simulink model "merge_activation"  (Simulink 8.2)
settings: Solver=ode1  StartTime=0.0  StopTime=Inf  FixedStep=0.001  RelTol=1e-3
PostLoadFcn:
  | , if any(exist('dsrtsu_mdlpostloadfcn', 'file') == [2, 3, 6]), try dsrtsu_mdlpostloadfcn('Execute', bdroot); catch fprintf('Error in PostLoadFcn (dsrtsu_mdlpostloadfcn) for model "%s":\n %s\n', bdroot, lasterr); end, end,
settings Model: DSRTSU_INTERNAL_RTI_VER=450  DSRTSU_INTERNAL_RTI_TYPE=rti1401  DSRTSU_INTERNAL_RTIFPGA=40  Creator=rushk1  LastModifiedBy=rushk1  BufferReuse=off
settings DataIOCC: SignalLoggingSaveFormat=Dataset
settings OptimizationCC: BlockReduction=off  OptimizeBlockIOStorage=off  BufferReuse=off  ExpressionFolding=off  ExpressionDepthLimit=128  LocalBlockOutputs=off
settings DebuggingCC: FcnCallInpInsideContextMsg=EnableAllAsError  StateNameClashWarn=none
settings HardwareCC: TargetHWDeviceType=Generic->Custom
settings RTWCC: SystemTargetFile=rti1401.tlc  MakeCommand=make_rti  TemplateMakefile=rti1401.tmf  Description=dSPACE DS1401 Hardware Platform  ProcessScript=rti1401_make_rtw_hook
settings STFCustomTargetCC: CodeReplacementLibrary=ANSI_C  ParMdlRefBuildCompliant=on  GeneratePreprocessorConditionals=Disable all  MatFileLogging=on  SystemTargetFile=rti1401.tlc
settings GRTTargetCC: CompOptLevelCompliant=off  ConcurrentExecutionCompliant=off  ExtModeMexFile=noextcomm
settings CustomProperty: DataType=RTWOptions_EnumType_C__Program Files_dSPACE RCPHIL 2014-B_MATLAB_RTI_RTI1401_TLC_rti1401_1InitialSimState  Value=RUN
settings EnumStrPairs: String=RUN

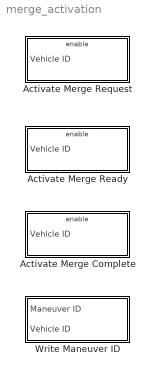
== system merge_activation ==
  Activate Merge Complete : Subsystem
  Activate Merge Ready : Subsystem
  Activate Merge Request : Subsystem
  Write Maneuver ID : Subsystem

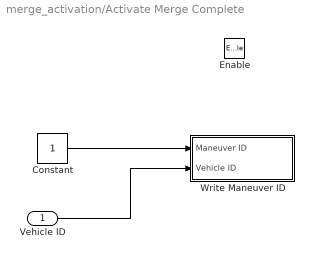
== system merge_activation/Activate Merge Complete ==
  Vehicle ID : Inport
  Enable : EnablePort
  Constant : Constant
  Write Maneuver ID : Subsystem
  wires:
  Constant/1 -> Write Maneuver ID/1(Maneuver ID)
  Vehicle ID/1 -> Write Maneuver ID/2(Vehicle ID)

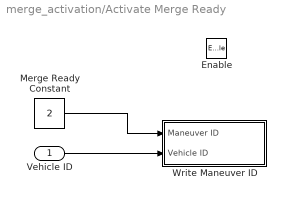
== system merge_activation/Activate Merge Ready ==
  Vehicle ID : Inport
  Enable : EnablePort
  Merge Ready Constant : Constant  Value=2
  Write Maneuver ID : Subsystem
  wires:
  Vehicle ID/1 -> Write Maneuver ID/2(Vehicle ID)
  Merge Ready Constant/1 -> Write Maneuver ID/1(Maneuver ID)

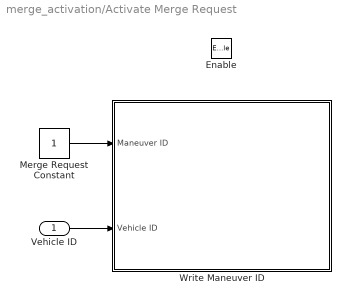
== system merge_activation/Activate Merge Request ==
  Vehicle ID : Inport
  Enable : EnablePort
  Merge Request Constant : Constant
  Write Maneuver ID : Subsystem
  wires:
  Merge Request Constant/1 -> Write Maneuver ID/1(Maneuver ID)
  Vehicle ID/1 -> Write Maneuver ID/2(Vehicle ID)

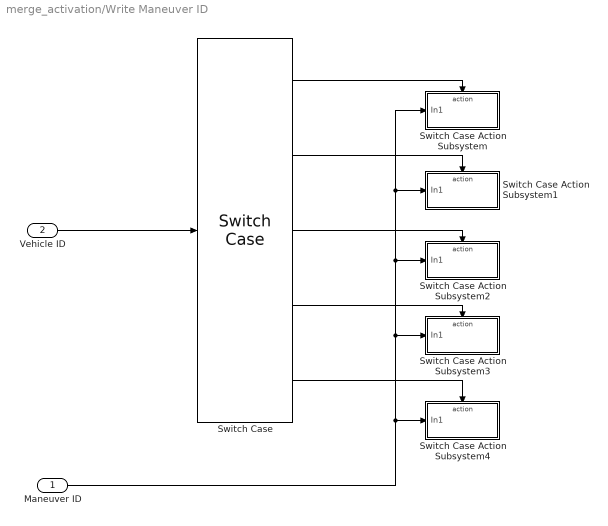
== system merge_activation/Write Maneuver ID ==
  Maneuver ID : Inport
  Vehicle ID : Inport  Port=2
  Switch Case : SwitchCase  CaseConditions={1,2,3,4,5}  ShowDefaultCase=off
  Switch Case Action Subsystem : Subsystem  TreatAsAtomicUnit=on
  Switch Case Action Subsystem1 : Subsystem  TreatAsAtomicUnit=on
  Switch Case Action Subsystem2 : Subsystem  TreatAsAtomicUnit=on
  Switch Case Action Subsystem3 : Subsystem  TreatAsAtomicUnit=on
  Switch Case Action Subsystem4 : Subsystem  TreatAsAtomicUnit=on
  wires:
  Switch Case/5 -> Switch Case Action Subsystem4/Action
  Switch Case/4 -> Switch Case Action Subsystem3/Action
  Switch Case/3 -> Switch Case Action Subsystem2/Action
  Switch Case/2 -> Switch Case Action Subsystem1/Action
  Switch Case/1 -> Switch Case Action Subsystem/Action
  Vehicle ID/1 -> Switch Case/1
  Maneuver ID/1 -> Switch Case Action Subsystem/1(In1), Switch Case Action Subsystem1/1(In1), Switch Case Action Subsystem2/1(In1), Switch Case Action Subsystem3/1(In1), Switch Case Action Subsystem4/1(In1)

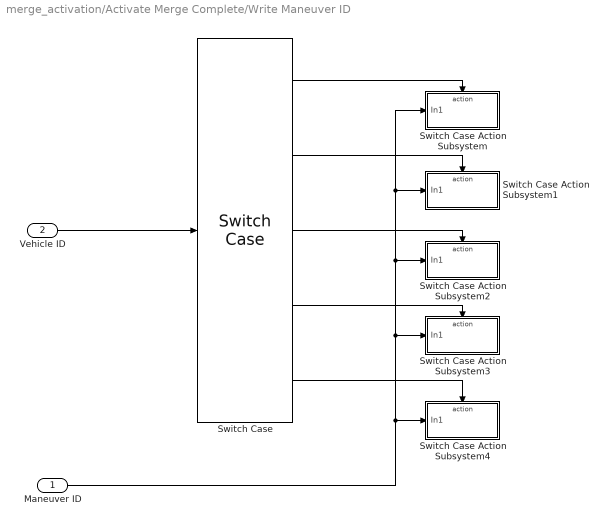
== system merge_activation/Activate Merge Complete/Write Maneuver ID ==
  Maneuver ID : Inport
  Vehicle ID : Inport  Port=2
  Switch Case : SwitchCase  CaseConditions={1,2,3,4,5}  ShowDefaultCase=off
  Switch Case Action Subsystem : Subsystem  TreatAsAtomicUnit=on
  Switch Case Action Subsystem1 : Subsystem  TreatAsAtomicUnit=on
  Switch Case Action Subsystem2 : Subsystem  TreatAsAtomicUnit=on
  Switch Case Action Subsystem3 : Subsystem  TreatAsAtomicUnit=on
  Switch Case Action Subsystem4 : Subsystem  TreatAsAtomicUnit=on
  wires:
  Switch Case/5 -> Switch Case Action Subsystem4/Action
  Switch Case/4 -> Switch Case Action Subsystem3/Action
  Switch Case/3 -> Switch Case Action Subsystem2/Action
  Switch Case/2 -> Switch Case Action Subsystem1/Action
  Switch Case/1 -> Switch Case Action Subsystem/Action
  Vehicle ID/1 -> Switch Case/1
  Maneuver ID/1 -> Switch Case Action Subsystem/1(In1), Switch Case Action Subsystem1/1(In1), Switch Case Action Subsystem2/1(In1), Switch Case Action Subsystem3/1(In1), Switch Case Action Subsystem4/1(In1)

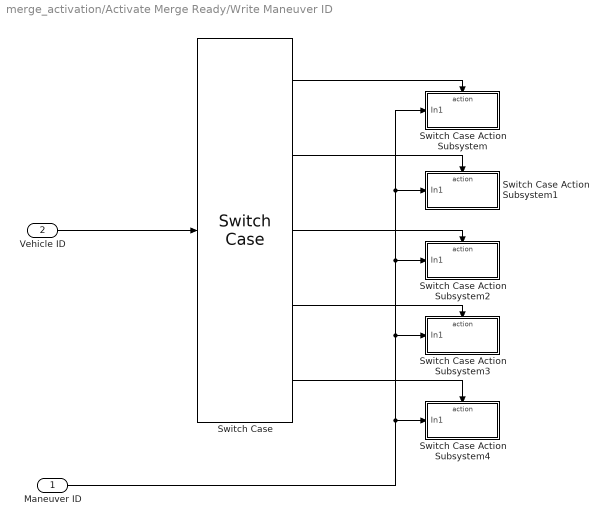
== system merge_activation/Activate Merge Ready/Write Maneuver ID ==
  Maneuver ID : Inport
  Vehicle ID : Inport  Port=2
  Switch Case : SwitchCase  CaseConditions={1,2,3,4,5}  ShowDefaultCase=off
  Switch Case Action Subsystem : Subsystem  TreatAsAtomicUnit=on
  Switch Case Action Subsystem1 : Subsystem  TreatAsAtomicUnit=on
  Switch Case Action Subsystem2 : Subsystem  TreatAsAtomicUnit=on
  Switch Case Action Subsystem3 : Subsystem  TreatAsAtomicUnit=on
  Switch Case Action Subsystem4 : Subsystem  TreatAsAtomicUnit=on
  wires:
  Switch Case/5 -> Switch Case Action Subsystem4/Action
  Switch Case/4 -> Switch Case Action Subsystem3/Action
  Switch Case/3 -> Switch Case Action Subsystem2/Action
  Switch Case/2 -> Switch Case Action Subsystem1/Action
  Switch Case/1 -> Switch Case Action Subsystem/Action
  Vehicle ID/1 -> Switch Case/1
  Maneuver ID/1 -> Switch Case Action Subsystem/1(In1), Switch Case Action Subsystem1/1(In1), Switch Case Action Subsystem2/1(In1), Switch Case Action Subsystem3/1(In1), Switch Case Action Subsystem4/1(In1)

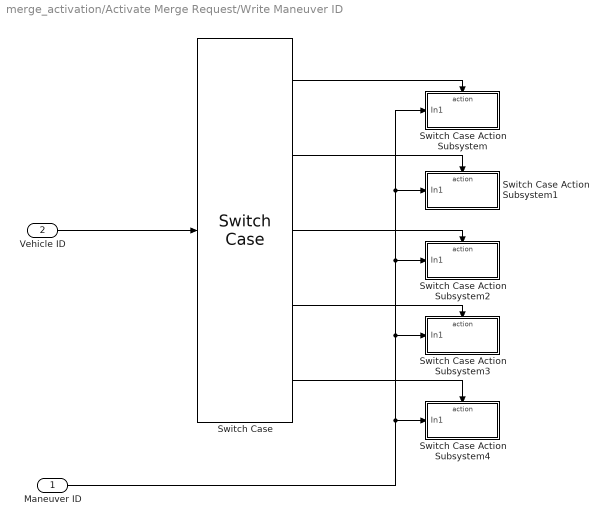
== system merge_activation/Activate Merge Request/Write Maneuver ID ==
  Maneuver ID : Inport
  Vehicle ID : Inport  Port=2
  Switch Case : SwitchCase  CaseConditions={1,2,3,4,5}  ShowDefaultCase=off
  Switch Case Action Subsystem : Subsystem  TreatAsAtomicUnit=on
  Switch Case Action Subsystem1 : Subsystem  TreatAsAtomicUnit=on
  Switch Case Action Subsystem2 : Subsystem  TreatAsAtomicUnit=on
  Switch Case Action Subsystem3 : Subsystem  TreatAsAtomicUnit=on
  Switch Case Action Subsystem4 : Subsystem  TreatAsAtomicUnit=on
  wires:
  Switch Case/5 -> Switch Case Action Subsystem4/Action
  Switch Case/4 -> Switch Case Action Subsystem3/Action
  Switch Case/3 -> Switch Case Action Subsystem2/Action
  Switch Case/2 -> Switch Case Action Subsystem1/Action
  Switch Case/1 -> Switch Case Action Subsystem/Action
  Vehicle ID/1 -> Switch Case/1
  Maneuver ID/1 -> Switch Case Action Subsystem/1(In1), Switch Case Action Subsystem1/1(In1), Switch Case Action Subsystem2/1(In1), Switch Case Action Subsystem3/1(In1), Switch Case Action Subsystem4/1(In1)

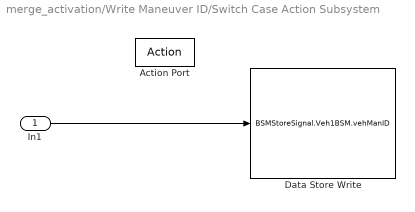
== system merge_activation/Write Maneuver ID/Switch Case Action Subsystem ==
  In1 : Inport
  Action Port : ActionPort
  Data Store Write : DataStoreWrite  DataStoreName=BSMStoreSignal  DataStoreElements=BSMStoreSignal.Veh1BSM.vehManID
  wires:
  In1/1 -> Data Store Write/1

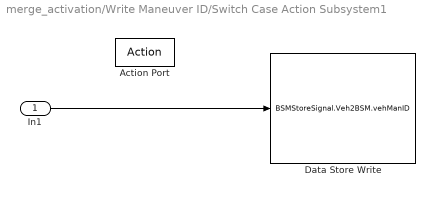
== system merge_activation/Write Maneuver ID/Switch Case Action Subsystem1 ==
  In1 : Inport
  Action Port : ActionPort
  Data Store Write : DataStoreWrite  DataStoreName=BSMStoreSignal  DataStoreElements=BSMStoreSignal.Veh2BSM.vehManID
  wires:
  In1/1 -> Data Store Write/1

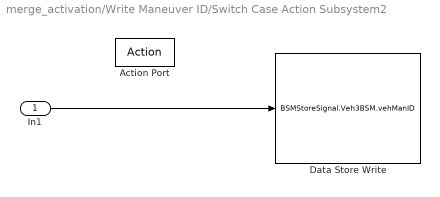
== system merge_activation/Write Maneuver ID/Switch Case Action Subsystem2 ==
  In1 : Inport
  Action Port : ActionPort
  Data Store Write : DataStoreWrite  DataStoreName=BSMStoreSignal  DataStoreElements=BSMStoreSignal.Veh3BSM.vehManID
  wires:
  In1/1 -> Data Store Write/1

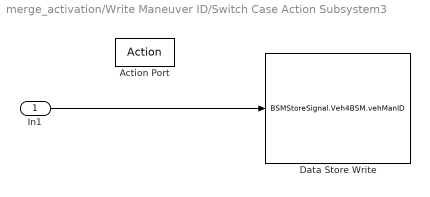
== system merge_activation/Write Maneuver ID/Switch Case Action Subsystem3 ==
  In1 : Inport
  Action Port : ActionPort
  Data Store Write : DataStoreWrite  DataStoreName=BSMStoreSignal  DataStoreElements=BSMStoreSignal.Veh4BSM.vehManID
  wires:
  In1/1 -> Data Store Write/1

== system merge_activation/Write Maneuver ID/Switch Case Action Subsystem4 ==
  In1 : Inport
  Action Port : ActionPort
  Data Store Write : DataStoreWrite  DataStoreName=BSMStoreSignal  DataStoreElements=BSMStoreSignal.Veh5BSM.vehManID
  wires:
  In1/1 -> Data Store Write/1

== system merge_activation/Activate Merge Complete/Write Maneuver ID/Switch Case Action Subsystem ==
  In1 : Inport
  Action Port : ActionPort
  Data Store Write : DataStoreWrite  DataStoreName=BSMStoreSignal  DataStoreElements=BSMStoreSignal.Veh1BSM.vehManID
  wires:
  In1/1 -> Data Store Write/1

== system merge_activation/Activate Merge Complete/Write Maneuver ID/Switch Case Action Subsystem1 ==
  In1 : Inport
  Action Port : ActionPort
  Data Store Write : DataStoreWrite  DataStoreName=BSMStoreSignal  DataStoreElements=BSMStoreSignal.Veh2BSM.vehManID
  wires:
  In1/1 -> Data Store Write/1

== system merge_activation/Activate Merge Complete/Write Maneuver ID/Switch Case Action Subsystem2 ==
  In1 : Inport
  Action Port : ActionPort
  Data Store Write : DataStoreWrite  DataStoreName=BSMStoreSignal  DataStoreElements=BSMStoreSignal.Veh3BSM.vehManID
  wires:
  In1/1 -> Data Store Write/1

== system merge_activation/Activate Merge Complete/Write Maneuver ID/Switch Case Action Subsystem3 ==
  In1 : Inport
  Action Port : ActionPort
  Data Store Write : DataStoreWrite  DataStoreName=BSMStoreSignal  DataStoreElements=BSMStoreSignal.Veh4BSM.vehManID
  wires:
  In1/1 -> Data Store Write/1

== system merge_activation/Activate Merge Complete/Write Maneuver ID/Switch Case Action Subsystem4 ==
  In1 : Inport
  Action Port : ActionPort
  Data Store Write : DataStoreWrite  DataStoreName=BSMStoreSignal  DataStoreElements=BSMStoreSignal.Veh5BSM.vehManID
  wires:
  In1/1 -> Data Store Write/1

== system merge_activation/Activate Merge Ready/Write Maneuver ID/Switch Case Action Subsystem ==
  In1 : Inport
  Action Port : ActionPort
  Data Store Write : DataStoreWrite  DataStoreName=BSMStoreSignal  DataStoreElements=BSMStoreSignal.Veh1BSM.vehManID
  wires:
  In1/1 -> Data Store Write/1

== system merge_activation/Activate Merge Ready/Write Maneuver ID/Switch Case Action Subsystem1 ==
  In1 : Inport
  Action Port : ActionPort
  Data Store Write : DataStoreWrite  DataStoreName=BSMStoreSignal  DataStoreElements=BSMStoreSignal.Veh2BSM.vehManID
  wires:
  In1/1 -> Data Store Write/1

== system merge_activation/Activate Merge Ready/Write Maneuver ID/Switch Case Action Subsystem2 ==
  In1 : Inport
  Action Port : ActionPort
  Data Store Write : DataStoreWrite  DataStoreName=BSMStoreSignal  DataStoreElements=BSMStoreSignal.Veh3BSM.vehManID
  wires:
  In1/1 -> Data Store Write/1

== system merge_activation/Activate Merge Ready/Write Maneuver ID/Switch Case Action Subsystem3 ==
  In1 : Inport
  Action Port : ActionPort
  Data Store Write : DataStoreWrite  DataStoreName=BSMStoreSignal  DataStoreElements=BSMStoreSignal.Veh4BSM.vehManID
  wires:
  In1/1 -> Data Store Write/1

== system merge_activation/Activate Merge Ready/Write Maneuver ID/Switch Case Action Subsystem4 ==
  In1 : Inport
  Action Port : ActionPort
  Data Store Write : DataStoreWrite  DataStoreName=BSMStoreSignal  DataStoreElements=BSMStoreSignal.Veh5BSM.vehManID
  wires:
  In1/1 -> Data Store Write/1

== system merge_activation/Activate Merge Request/Write Maneuver ID/Switch Case Action Subsystem ==
  In1 : Inport
  Action Port : ActionPort
  Data Store Write : DataStoreWrite  DataStoreName=BSMStoreSignal  DataStoreElements=BSMStoreSignal.Veh1BSM.vehManID
  wires:
  In1/1 -> Data Store Write/1

== system merge_activation/Activate Merge Request/Write Maneuver ID/Switch Case Action Subsystem1 ==
  In1 : Inport
  Action Port : ActionPort
  Data Store Write : DataStoreWrite  DataStoreName=BSMStoreSignal  DataStoreElements=BSMStoreSignal.Veh2BSM.vehManID
  wires:
  In1/1 -> Data Store Write/1

== system merge_activation/Activate Merge Request/Write Maneuver ID/Switch Case Action Subsystem2 ==
  In1 : Inport
  Action Port : ActionPort
  Data Store Write : DataStoreWrite  DataStoreName=BSMStoreSignal  DataStoreElements=BSMStoreSignal.Veh3BSM.vehManID
  wires:
  In1/1 -> Data Store Write/1

== system merge_activation/Activate Merge Request/Write Maneuver ID/Switch Case Action Subsystem3 ==
  In1 : Inport
  Action Port : ActionPort
  Data Store Write : DataStoreWrite  DataStoreName=BSMStoreSignal  DataStoreElements=BSMStoreSignal.Veh4BSM.vehManID
  wires:
  In1/1 -> Data Store Write/1

== system merge_activation/Activate Merge Request/Write Maneuver ID/Switch Case Action Subsystem4 ==
  In1 : Inport
  Action Port : ActionPort
  Data Store Write : DataStoreWrite  DataStoreName=BSMStoreSignal  DataStoreElements=BSMStoreSignal.Veh5BSM.vehManID
  wires:
  In1/1 -> Data Store Write/1
